simulink model "continuousHopfieldNetwork"  (R2017a)
settings: Solver=ode1  StartTime=0.0  StopTime=10  FixedStep=dt  RelTol=1e-3  EnableMultiTasking=on
undefined symbols (not defined in the file or in its folder): ib, lambda, T, v0
settings Model: Creator=Lucas  LastModifiedBy=Lucas
settings DataIOCC: SaveFormat=Array
settings OptimizationCC: LifeSpan=inf
settings DebuggingCC: SFUnexpectedBacktrackingDiag=warning  SFNoUnconditionalDefaultTransitionDiag=warning  SFExecutionAtInitializationDiag=none
settings GRTTargetCC: TargetLangStandard=C89/C90 (ANSI)  GeneratePreprocessorConditionals=Disable all
settings ConfigComp: CovMetricSettings=dw  CovHtmlReporting=on  CovSaveCumulativeToWorkspaceVar=on  CovSaveSingleToWorkspaceVar=on  CovExternalEMLEnable=off

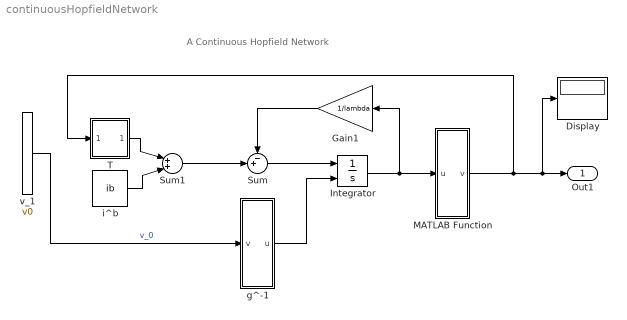
== system continuousHopfieldNetwork ==
  note: A Continuous Hopfield Network
  Display : Display
  Gain1 : Gain  Gain=1/lambda
  Integrator : Integrator  InitialConditionSource=external
  MATLAB Function : MATLAB Function  TreatAsAtomicUnit=on
  Sum : Sum  Inputs=-+|
  Sum1 : Sum  Inputs=|++|
  T : Subsystem
      mask Display: disp('T')
  g^-1 : MATLAB Function  TreatAsAtomicUnit=on
  i^b : Constant  Value=ib
  v_1 : Constant  Value=v0
      mask Display: disp('')
  Out1 : Outport
  wires:
  v_1/1 -> g^-1/1(v)  "v_0"
  Integrator/1 -> MATLAB Function/1(u), Gain1/1
  MATLAB Function/1(v) -> Out1/1, Display/1, T/1(In1)
  g^-1/1(u) -> Integrator/2
  Sum1/1 -> Sum/2
  Sum/1 -> Integrator/1
  Gain1/1 -> Sum/1
  T/1(Out1) -> Sum1/1
  i^b/1 -> Sum1/2

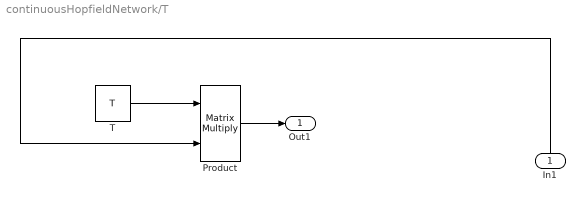
== system continuousHopfieldNetwork/T ==
  In1 : Inport
  Product : Product  Multiplication=Matrix(*)
  T : Constant  Value=T
  Out1 : Outport
  wires:
  Product/1 -> Out1/1
  T/1 -> Product/1
  In1/1 -> Product/2

== matlab function continuousHopfieldNetwork/g^-1 ==
  data: v input; u output
function u = mySigmoidInverse(v)
    u0 = 0.3;
    
    u = (u0/2)*log(v./(1-v));
end

== matlab function continuousHopfieldNetwork/MATLAB Function ==
  data: u input; v output
function v = mySigmoid(u)
u0 = 0.3;

v = 0.5*(1+tanh(u./u0));

end
